simulink model "MIL4L3_SW6_V1_20220211"  (R2018b)
settings: Solver=FixedStepAuto  StartTime=0.0  StopTime=inf  FixedStep=0.001  RelTol=1e-3
PreLoadFcn:
  | A0_MILtest;
undefined symbols (not defined in the file or in its folder): Clb_ICADirect_LaneDisp_StateFive, Clb_ICADirect_LaneDisp_StateFour, Clb_ICADirect_LaneDisp_StateOne, Clb_ICADirect_LaneDisp_StateThree, Clb_ICADirect_LaneDisp_StateTwo, Clb_ICADirect_LaneDisp_StateZero, Clb_ICADirect_LaneDispSW, Clb_ICADirect_TrnLghtsCom_Switch, Clb_ICADirect_TrnLghtsCom_Value, Clb_ICADirect_TrnLghtsCrtl_Inhb, IMAP_Clb_ACU_Driver_Belt, IMAP_Clb_ACU_Driver_Belt_Over, IMAP_Clb_ACU_Passenger_Belt, IMAP_Clb_ACU_Passenger_Belt_Over, IMAP_Clb_ACU_RearLeft_Belt, IMAP_Clb_ACU_RearLeft_Belt_Over, IMAP_Clb_ACU_RearMiddle_Belt, IMAP_Clb_ACU_RearMiddle_Belt_Over, IMAP_Clb_ACU_RearRight_Belt, IMAP_Clb_ACU_RearRight_Belt_Over, IMAP_Clb_AEB_Switch, IMAP_Clb_AEB_Switch_Over, IMAP_Clb_ALC_TLC_Mode, IMAP_Clb_ALC_TLC_Mode_Over, IMAP_Clb_BCM_Battery_Voltage, IMAP_Clb_BCM_Battery_Voltage_Over, IMAP_Clb_BCM_BrakeLamp_State, IMAP_Clb_BCM_BrakeLamp_State_Over, IMAP_Clb_BCM_CHMSL_Status, IMAP_Clb_BCM_CHMSL_Status_Over, IMAP_Clb_BCM_Door_Lock_State, IMAP_Clb_BCM_Door_Lock_State_Over, IMAP_Clb_BCM_FrontWiper_State, IMAP_Clb_BCM_FrontWiper_State_Over, IMAP_Clb_BCM_FrontWiper_Switch, IMAP_Clb_BCM_FrontWiper_Switch_Over, IMAP_Clb_BCM_HazardLamp, IMAP_Clb_BCM_HazardLamp_Over, IMAP_Clb_BCM_HazardLamp_Switch, IMAP_Clb_BCM_HazardLamp_Switch_Over, IMAP_Clb_BCM_HighBeam_State, IMAP_Clb_BCM_HighBeam_State_Over, IMAP_Clb_BCM_Ignition_State, IMAP_Clb_BCM_Ignition_State_Over, IMAP_Clb_BCM_IHBC_Enabled, IMAP_Clb_BCM_IHBC_Enabled_Over, IMAP_Clb_BCM_Left_Light, IMAP_Clb_BCM_Left_Light_Over, IMAP_Clb_BCM_LeftTurn_Switch, IMAP_Clb_BCM_LeftTurn_Switch_Over, IMAP_Clb_BCM_LF_Door_State, IMAP_Clb_BCM_LF_Door_State_Over, IMAP_Clb_BCM_LowBeam_State, IMAP_Clb_BCM_LowBeam_State_Over, IMAP_Clb_BCM_LR_Door_State, IMAP_Clb_BCM_LR_Door_State_Over, IMAP_Clb_BCM_RF_Door_State, IMAP_Clb_BCM_RF_Door_State_Over, IMAP_Clb_BCM_Right_Light, IMAP_Clb_BCM_Right_Light_Over ... (+547)
libraries: CarMaker4SL x2153, simulink x292, dspstat3 x3, canmsglib x2, simulink_extras x1
(part 7 of 52)

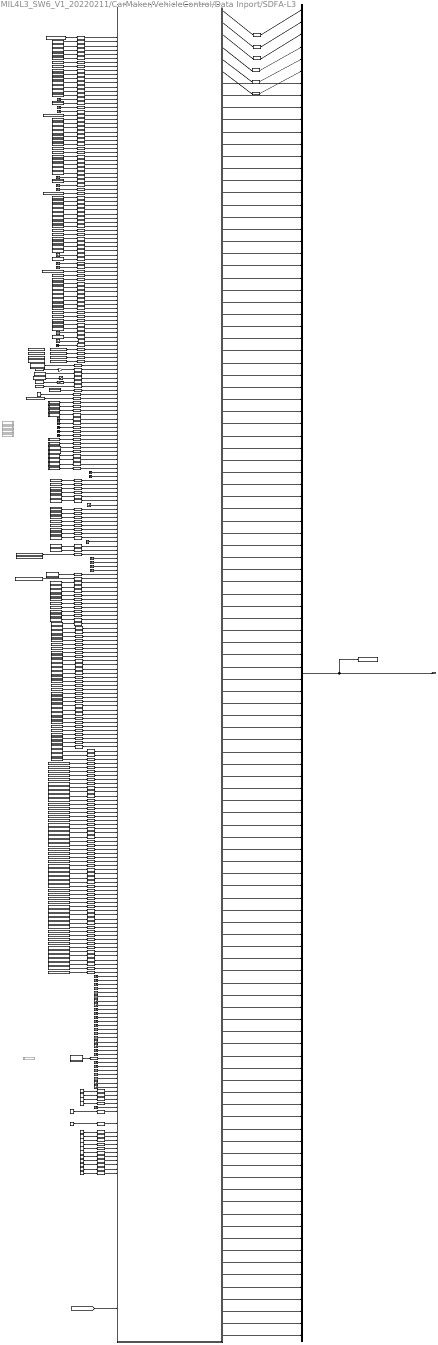
== system MIL4L3_SW6_V1_20220211/CarMaker/VehicleControl/Data Inport/SDFA-L3 ==
  note: SDFA-L3
  ACCEL_LONGI_CALIB2 : Saturate  UpperLimit=40.92  LowerLimit=-40.96
  BusCreator3 : BusCreator  Inputs=110
  CIPV_ID1 : Subsystem
  Constant{1..8,10..14,16..19} (17 alike) : Constant  Value=0
  Constant9 : Constant
  Data Type  Conversion{1..4,6,8..12,508} (11 alike) : DataTypeConversion
  Data Type Conversion{,1..94,98,118,128..129,131..251,253..265,267} (234 alike) : DataTypeConversion
  Define CM Dict : CarMaker4SL/Define CM Dict  xname=User.IO.Out.CRFLstatus  xmono=off  xtype=Double4  xdvaplace=None  xnstates=0  xfirststate=0  xinitial=0
  Define CM Dict1 : CarMaker4SL/Define CM Dict  xname=User.IO.Out.CRFRstatus  xmono=off  xtype=Double4  xdvaplace=None  xnstates=0  xfirststate=0  xinitial=0
  Define CM Dict3 : CarMaker4SL/Define CM Dict  xname=User.IO.Out.CRRLstatus  xmono=off  xtype=Double4  xdvaplace=None  xnstates=0  xfirststate=0  xinitial=0
  Define CM Dict4 : CarMaker4SL/Define CM Dict  xname=User.IO.Out.CRRRstatus  xmono=off  xtype=Double4  xdvaplace=None  xnstates=0  xfirststate=0  xinitial=0
  Define CM Dict7 : CarMaker4SL/Define CM Dict  xname=User.IO.Out.IFCState  xmono=off  xtype=Double4  xdvaplace=IO_Out  xnstates=0  xfirststate=0  xinitial=9
  Gain10 : Gain  Gain=3.6
  Ground{,1..41,43..46,52,56..61} (53 alike) : Ground
  Lateral_acceleration1 : CarMaker4SL/Read CM Dict  xname=Car.ay  xsync=off
  Lateral_acceleration2 : CarMaker4SL/Read CM Dict  xname=User.IO.Out.CRFLstatus  xsync=off
  Lateral_acceleration3 : CarMaker4SL/Read CM Dict  xname=User.IO.Out.CRFRstatus  xsync=off
  Lateral_acceleration4 : CarMaker4SL/Read CM Dict  xname=User.IO.Out.CRRLstatus  xsync=off
  Lateral_acceleration5 : CarMaker4SL/Read CM Dict  xname=User.IO.Out.CRRRstatus  xsync=off
  Read CM Dict : CarMaker4SL/Read CM Dict  xname=User.IO.Out.IFC_Line01_CurvChange  xsync=off
  Read CM Dict1 : CarMaker4SL/Read CM Dict  xname=User.IO.Out.NumberOfObjects_S3  xsync=off
  Read CM Dict10 : CarMaker4SL/Read CM Dict  xname=User.IO.Out.IFC_Line01_Dy  xsync=off
  Read CM Dict11 : CarMaker4SL/Read CM Dict  xname=User.IO.Out.IFC_Line01_ExistProb  xsync=off
  Read CM Dict12 : CarMaker4SL/Read CM Dict  xname=User.IO.Out.IFC_Line01_MeasureType  xsync=off
  Read CM Dict13 : CarMaker4SL/Read CM Dict  xname=User.IO.Out.IFC_Line01_Type  xsync=off
  Read CM Dict14 : CarMaker4SL/Read CM Dict  xname=User.IO.Out.IFC_Line01_LineID  xsync=off
  Read CM Dict15 : CarMaker4SL/Read CM Dict  xname=User.IO.Out.IFC_Line01_TypeConf  xsync=off
  Read CM Dict16 : CarMaker4SL/Read CM Dict  xname=User.IO.Out.IFC_Line01_ColorClass  xsync=off
  Read CM Dict17 : CarMaker4SL/Read CM Dict  xname=User.IO.Out.IFC_Line01_DxStart  xsync=off
  Read CM Dict18 : CarMaker4SL/Read CM Dict  xname=User.IO.Out.IFC_Line01_DxEnd  xsync=off
  Read CM Dict19 : CarMaker4SL/Read CM Dict  xname=User.IO.Out.IFC_Line01_LineWidth  xsync=off
  Read CM Dict2 : CarMaker4SL/Read CM Dict  xname=User.IO.Out.IFCState  xsync=off
  Read CM Dict20 : CarMaker4SL/Read CM Dict  xname=User.IO.Out.IFC_Line02_CurvChange  xsync=off
  Read CM Dict21 : CarMaker4SL/Read CM Dict  xname=User.IO.Out.IFC_Line02_Curv  xsync=off
  Read CM Dict22 : CarMaker4SL/Read CM Dict  xname=User.IO.Out.IFC_Line02_HeadingAngle  xsync=off
  Read CM Dict23 : CarMaker4SL/Read CM Dict  xname=User.IO.Out.IFC_Line02_Dy  xsync=off
  Read CM Dict24 : CarMaker4SL/Read CM Dict  xname=User.IO.Out.IFC_Line02_ExistProb  xsync=off
  Read CM Dict25 : CarMaker4SL/Read CM Dict  xname=Car.ax  xsync=off
  Read CM Dict26 : CarMaker4SL/Read CM Dict  xname=Car.v  xsync=off
  Read CM Dict27 : CarMaker4SL/Read CM Dict  xname=Steer.WhlAng  xsync=off
  Read CM Dict28 : CarMaker4SL/Read CM Dict  xname=User.IO.Out.IFC_Line02_MeasureType  xsync=off
  Read CM Dict29 : CarMaker4SL/Read CM Dict  xname=User.IO.Out.IFC_Line02_Type  xsync=off
  Read CM Dict3 : CarMaker4SL/Read CM Dict  xname=User.IO.Out.NumberOfObjects_S0  xsync=off
  Read CM Dict30 : CarMaker4SL/Read CM Dict  xname=User.IO.Out.IFC_Line02_LineID  xsync=off
  Read CM Dict31 : CarMaker4SL/Read CM Dict  xname=User.IO.Out.IFC_Line02_TypeConf  xsync=off
  Read CM Dict32 : CarMaker4SL/Read CM Dict  xname=User.IO.Out.IFC_Line02_ColorClass  xsync=off
  Read CM Dict33 : CarMaker4SL/Read CM Dict  xname=User.IO.Out.IFC_Line02_DxStart  xsync=off
  Read CM Dict34 : CarMaker4SL/Read CM Dict  xname=User.IO.Out.IFC_Line02_DxEnd  xsync=off
  Read CM Dict35 : CarMaker4SL/Read CM Dict  xname=User.IO.Out.IFC_Line02_LineWidth  xsync=off
  Read CM Dict36 : CarMaker4SL/Read CM Dict  xname=User.IO.Out.IFC_Line03_CurvChange  xsync=off
  Read CM Dict37 : CarMaker4SL/Read CM Dict  xname=User.IO.Out.IFC_Line03_Curv  xsync=off
  Read CM Dict38 : CarMaker4SL/Read CM Dict  xname=User.IO.Out.IFC_Line03_HeadingAngle  xsync=off
  Read CM Dict39 : CarMaker4SL/Read CM Dict  xname=User.IO.Out.IFC_Line03_Dy  xsync=off
  Read CM Dict4 : CarMaker4SL/Read CM Dict  xname=User.IO.Out.NumberOfObjects_S1  xsync=off
  Read CM Dict40 : CarMaker4SL/Read CM Dict  xname=User.IO.Out.IFC_Line03_ExistProb  xsync=off
  Read CM Dict41 : CarMaker4SL/Read CM Dict  xname=User.IO.Out.IFC_Line03_MeasureType  xsync=off
  Read CM Dict42 : CarMaker4SL/Read CM Dict  xname=User.IO.Out.IFC_Line03_Type  xsync=off
  Read CM Dict43 : CarMaker4SL/Read CM Dict  xname=User.IO.Out.IFC_Line03_LineID  xsync=off
  Read CM Dict44 : CarMaker4SL/Read CM Dict  xname=User.IO.Out.IFC_Line03_TypeConf  xsync=off
  Read CM Dict45 : CarMaker4SL/Read CM Dict  xname=User.IO.Out.IFC_Line03_ColorClass  xsync=off
  Read CM Dict46 : CarMaker4SL/Read CM Dict  xname=User.IO.Out.IFC_Line03_DxStart  xsync=off
  Read CM Dict47 : CarMaker4SL/Read CM Dict  xname=User.IO.Out.IFC_Line03_DxEnd  xsync=off
  Read CM Dict48 : CarMaker4SL/Read CM Dict  xname=User.IO.Out.IFC_Line03_LineWidth  xsync=off
  Read CM Dict49 : CarMaker4SL/Read CM Dict  xname=User.IO.Out.IFC_Line04_CurvChange  xsync=off
  Read CM Dict5 : CarMaker4SL/Read CM Dict  xname=User.IO.Out.NumberOfObjects_S2  xsync=off
  Read CM Dict50 : CarMaker4SL/Read CM Dict  xname=User.IO.Out.IFC_Line04_Curv  xsync=off
  Read CM Dict51 : CarMaker4SL/Read CM Dict  xname=User.IO.Out.IFC_Line04_HeadingAngle  xsync=off
  Read CM Dict52 : CarMaker4SL/Read CM Dict  xname=User.IO.Out.IFC_Line04_Dy  xsync=off
  Read CM Dict53 : CarMaker4SL/Read CM Dict  xname=User.IO.Out.IFC_Line04_ExistProb  xsync=off
  Read CM Dict54 : CarMaker4SL/Read CM Dict  xname=User.IO.Out.IFC_Line04_MeasureType  xsync=off
  Read CM Dict55 : CarMaker4SL/Read CM Dict  xname=User.IO.Out.IFC_Line04_Type  xsync=off
  Read CM Dict56 : CarMaker4SL/Read CM Dict  xname=User.IO.Out.IFC_Line04_LineID  xsync=off
  Read CM Dict57 : CarMaker4SL/Read CM Dict  xname=User.IO.Out.IFC_Line04_TypeConf  xsync=off
  Read CM Dict58 : CarMaker4SL/Read CM Dict  xname=User.IO.Out.IFC_Line04_ColorClass  xsync=off
  Read CM Dict59 : CarMaker4SL/Read CM Dict  xname=User.IO.Out.IFC_Line04_DxStart  xsync=off
  Read CM Dict6 : CarMaker4SL/Read CM Dict  xname=User.IO.Out.NumberOfObj  xsync=off
  Read CM Dict60 : CarMaker4SL/Read CM Dict  xname=User.IO.Out.IFC_Line04_DxEnd  xsync=off
  Read CM Dict61 : CarMaker4SL/Read CM Dict  xname=User.IO.Out.IFC_Line04_LineWidth  xsync=off
  Read CM Dict62 : CarMaker4SL/Read CM Dict  xname=User.IO.Out.ObjCount  xsync=off
  Read CM Dict8 : CarMaker4SL/Read CM Dict  xname=User.IO.Out.IFC_Line01_Curv  xsync=off
  Read CM Dict9 : CarMaker4SL/Read CM Dict  xname=User.IO.Out.IFC_Line01_HeadingAngle  xsync=off
  SDFA-L3 : ModelReference  ModelNameDialog=SDFA_SW6_1_MIL.slxp  ModelReferenceVersion=1.248  CopyOfModelProtected=on
  Saturation3 : Saturate  UpperLimit=780  LowerLimit=-780
  Subsystem : Subsystem
  Subsystem1 : Subsystem
  Subsystem10 : Subsystem
  Subsystem100 : Subsystem
  Subsystem103 : Subsystem
  Subsystem107 : Subsystem
  Subsystem108 : Subsystem
  Subsystem109 : Subsystem
  Subsystem11 : Subsystem
  Subsystem110 : Subsystem
  Subsystem111 : Subsystem
  Subsystem112 : Subsystem
  Subsystem113 : Subsystem
  Subsystem114 : Subsystem
  Subsystem115 : Subsystem
  Subsystem116 : Subsystem
  Subsystem117 : Subsystem
  Subsystem118 : Subsystem
  Subsystem119 : Subsystem
  Subsystem12 : Subsystem
  Subsystem120 : Subsystem
  Subsystem14 : Subsystem
  Subsystem149 : Subsystem
  Subsystem150 : Subsystem
  Subsystem160 : Subsystem
  Subsystem171 : Subsystem
  Subsystem174 : Subsystem
  Subsystem175 : Subsystem
  Subsystem176 : Subsystem
  Subsystem177 : Subsystem
  Subsystem178 : Subsystem
  Subsystem179 : Subsystem
  Subsystem180 : Subsystem
  Subsystem181 : Subsystem
  Subsystem182 : Subsystem
  Subsystem183 : Subsystem
  Subsystem184 : Subsystem
  Subsystem185 : Subsystem
  Subsystem186 : Subsystem
  Subsystem187 : Subsystem
  Subsystem188 : Subsystem
  Subsystem189 : Subsystem
  Subsystem190 : Subsystem
  Subsystem191 : Subsystem
  Subsystem192 : Subsystem
  Subsystem193 : Subsystem
  Subsystem194 : Subsystem
  Subsystem195 : Subsystem
  Subsystem196 : Subsystem
  Subsystem197 : Subsystem
  Subsystem198 : Subsystem
  Subsystem199 : Subsystem
  Subsystem2 : Subsystem
  Subsystem20 : Subsystem
  Subsystem200 : Subsystem
  Subsystem201 : Subsystem
  Subsystem202 : Subsystem
  Subsystem203 : Subsystem
  Subsystem204 : Subsystem
  Subsystem205 : Subsystem
  Subsystem206 : Subsystem
  Subsystem208 : Subsystem
  Subsystem209 : Subsystem
  Subsystem210 : Subsystem
  Subsystem211 : Subsystem
  Subsystem212 : Subsystem
  Subsystem214 : Subsystem
  Subsystem215 : Subsystem
  Subsystem216 : Subsystem
  Subsystem217 : Subsystem
  Subsystem218 : Subsystem
  Subsystem219 : Subsystem
  Subsystem220 : Subsystem
  Subsystem221 : Subsystem
  Subsystem222 : Subsystem
  Subsystem223 : Subsystem
  Subsystem224 : Subsystem
  Subsystem225 : Subsystem
  Subsystem226 : Subsystem
  Subsystem227 : Subsystem
  Subsystem228 : Subsystem
  Subsystem230 : Subsystem  Commented=on
  Subsystem232 : Subsystem
  Subsystem239 : Subsystem  Commented=on
  Subsystem255 : Subsystem
  Subsystem261 : Subsystem  Commented=on
  Subsystem272 : Subsystem  Commented=on
  Subsystem283 : Subsystem
  Subsystem3 : Subsystem
  Subsystem4 : Subsystem
  Subsystem40 : Subsystem
  Subsystem41 : Subsystem  Commented=on
  Subsystem46 : Subsystem
  Subsystem47 : Subsystem
  Subsystem48 : Subsystem
  Subsystem49 : Subsystem
  Subsystem5 : Subsystem
  Subsystem50 : Subsystem
  Subsystem51 : Subsystem
  Subsystem52 : Subsystem
  Subsystem53 : Subsystem
  Subsystem54 : Subsystem
  Subsystem55 : Subsystem
  Subsystem56 : Subsystem
  Subsystem57 : Subsystem
  Subsystem58 : Subsystem
  Subsystem59 : Subsystem
  Subsystem6 : Subsystem
  Subsystem61 : Subsystem
  Subsystem66 : Subsystem
  Subsystem67 : Subsystem
  Subsystem68 : Subsystem
  Subsystem69 : Subsystem
  Subsystem7 : Subsystem
  Subsystem70 : Subsystem
  Subsystem71 : Subsystem
  Subsystem72 : Subsystem
  Subsystem73 : Subsystem
  Subsystem74 : Subsystem
  Subsystem75 : Subsystem
  Subsystem76 : Subsystem
  Subsystem77 : Subsystem
  Subsystem78 : Subsystem
  Subsystem79 : Subsystem
  Subsystem8 : Subsystem
  Subsystem81 : Subsystem
  Subsystem85 : Subsystem
  Subsystem86 : Subsystem
  Subsystem87 : Subsystem
  Subsystem88 : Subsystem
  Subsystem89 : Subsystem
  Subsystem9 : Subsystem
  Subsystem90 : Subsystem
  Subsystem91 : Subsystem
  Subsystem92 : Subsystem
  Subsystem93 : Subsystem
  Subsystem94 : Subsystem
  Subsystem95 : Subsystem
  Subsystem96 : Subsystem
  Subsystem97 : Subsystem
  Subsystem98 : Subsystem
  To Workspace : ToWorkspace  VariableName=SDFAOUTPUT  SaveFormat=Timeseries  SampleTime=-1
  SDFAL3 : Outport
  wires:
  BusCreator3/1 -> To Workspace/1, SDFAL3/1
  SDFA-L3/1 -> Data Type  Conversion8/1
  SDFA-L3/6 -> Data Type  Conversion4/1
  Data Type  Conversion10/1 -> BusCreator3/3  "SDFAve_d_sen_sta_RF_radar"
  SDFA-L3/2 -> Data Type  Conversion9/1
  Data Type  Conversion9/1 -> BusCreator3/2  "SDFAve_d_sen_sta_LF_radar"
  Data Type  Conversion8/1 -> BusCreator3/1  "SDFAve_d_sensor_status"
  Data Type  Conversion11/1 -> BusCreator3/4  "SDFAve_d_sen_sta_LB_radar"
  Data Type  Conversion12/1 -> BusCreator3/5  "SDFAve_d_sen_sta_RB_radar"
  SDFA-L3/3 -> Data Type  Conversion10/1
  SDFA-L3/4 -> Data Type  Conversion11/1
  SDFA-L3/5 -> Data Type  Conversion12/1
  Lateral_acceleration2/1 -> Data Type Conversion131/1
  Lateral_acceleration3/1 -> Data Type Conversion132/1
  Lateral_acceleration4/1 -> Data Type Conversion133/1
  Lateral_acceleration5/1 -> Data Type Conversion134/1
  Data Type Conversion131/1 -> SDFA-L3/77
  Data Type Conversion132/1 -> SDFA-L3/78
  Data Type Conversion133/1 -> SDFA-L3/79
  Data Type Conversion134/1 -> SDFA-L3/80
  Data Type  Conversion4/1 -> BusCreator3/6  "SDFAve_d_fusion_status"
  Data Type Conversion149/1 -> SDFA-L3/12  "LFtar_ExistenceProbability"
  Data Type Conversion145/1 -> SDFA-L3/8  "LFtar_Yacceleration"
  Data Type Conversion148/1 -> SDFA-L3/11  "LFtar_Orientation"
  Data Type Conversion186/1 -> SDFA-L3/51  "LBtar_Class"
  Data Type Conversion139/1 -> SDFA-L3/2  "LFtar_id"
  Data Type Conversion206/1 -> SDFA-L3/73  "RBtar_ObjectInfo"
  Data Type Conversion150/1 -> SDFA-L3/13  "LFtar_Class"
  Data Type Conversion178/1 -> SDFA-L3/44  "LBtar_Yvelocity"
  Data Type Conversion179/1 -> SDFA-L3/45  "LBtar_Xacceleration"
  Data Type Conversion177/1 -> SDFA-L3/43  "LBtar_Xvelocity"
  Data Type Conversion167/1 -> SDFA-L3/32  "RFtar_Class"
  Data Type Conversion187/1 -> SDFA-L3/52  "LBtar_ReferencePoint"
  Data Type Conversion151/1 -> SDFA-L3/14  "LFtar_ReferencePoint"
  Data Type Conversion165/1 -> SDFA-L3/30  "RFtar_Orientation"
  Data Type Conversion147/1 -> SDFA-L3/10  "LFtar_Length"
  Data Type Conversion164/1 -> SDFA-L3/29  "RFtar_Length"
  Data Type Conversion163/1 -> SDFA-L3/28  "RFtar_Width"
  Data Type Conversion162/1 -> SDFA-L3/27  "RFtar_Yacceleration"
  Data Type Conversion161/1 -> SDFA-L3/26  "RFtar_Xacceleration"
  Data Type Conversion170/1 -> SDFA-L3/36  "RFtar_ClassHighestProb"
  Data Type Conversion169/1 -> SDFA-L3/35  "RFtar_ObjectInfo"
  Data Type Conversion188/1 -> SDFA-L3/54  "LBtar_ObjectInfo"
  Data Type Conversion193/1 -> SDFA-L3/61  "RBtar_Ypos"
  Data Type Conversion191/1 -> SDFA-L3/58  "RBtar_number"
  Data Type Conversion194/1 -> SDFA-L3/60  "RBtar_Xpos"
  Data Type Conversion143/1 -> SDFA-L3/6  "LFtar_Yvelocity"
  Subsystem47/1(LFtar_Xpos) -> Data Type Conversion140/1  "LFtar_Xpos"
  Data Type Conversion158/1 -> SDFA-L3/16  "LFtar_ObjectInfo"
  Subsystem46/1(LFtar_id) -> Data Type Conversion139/1  "LFtar_id"
  Data Type Conversion138/1 -> SDFA-L3/1  "LFtar_number"
  Data Type Conversion181/1 -> SDFA-L3/47  "LBtar_Width"
  Data Type Conversion184/1 -> SDFA-L3/50  "LBtar_ExistenceProbability"
  Data Type Conversion160/1 -> SDFA-L3/25  "RFtar_Yvelocity"
  Data Type Conversion197/1 -> SDFA-L3/63  "RBtar_Yvelocity"
  Data Type Conversion200/1 -> SDFA-L3/65  "RBtar_Yacceleration"
  Data Type Conversion182/1 -> SDFA-L3/48  "LBtar_Length"
  Data Type Conversion199/1 -> SDFA-L3/66  "RBtar_Width"
  Data Type Conversion203/1 -> SDFA-L3/69  "RBtar_ExistenceProbability"
  Data Type Conversion202/1 -> SDFA-L3/68  "RBtar_Orientation"
  Data Type Conversion189/1 -> SDFA-L3/55  "LBtar_ClassHighestProb"
  Data Type Conversion144/1 -> SDFA-L3/7  "LFtar_Xacceleration"
  Data Type Conversion140/1 -> SDFA-L3/3  "LFtar_Xpos"
  Data Type Conversion168/1 -> SDFA-L3/33  "RFtar_ReferencePoint"
  Data Type Conversion192/1 -> SDFA-L3/59  "RBtar_id"
  Data Type Conversion171/1 -> SDFA-L3/38  "RFtar_timestamp"
  Data Type Conversion208/1 -> SDFA-L3/74  "RBtar_ClassHighestProb"
  Data Type Conversion176/1 -> SDFA-L3/42  "LBtar_Ypos"
  Data Type Conversion172/1 -> SDFA-L3/39  "LBtar_number"
  Data Type Conversion142/1 -> SDFA-L3/5  "LFtar_Xvelocity"
  Data Type Conversion141/1 -> SDFA-L3/4  "LFtar_Ypos"
  Data Type Conversion166/1 -> SDFA-L3/31  "RFtar_ExistenceProbability"
  Data Type Conversion173/1 -> SDFA-L3/40  "LBtar_id"
  Data Type Conversion175/1 -> SDFA-L3/41  "LBtar_Xpos"
  Data Type Conversion201/1 -> SDFA-L3/67  "RBtar_Length"
  Data Type Conversion205/1 -> SDFA-L3/70  "RBtar_Class"
  Data Type Conversion204/1 -> SDFA-L3/71  "RBtar_ReferencePoint"
  Data Type Conversion152/1 -> SDFA-L3/19  "LFtar_timestamp"
  Data Type Conversion198/1 -> SDFA-L3/64  "RBtar_Xacceleration"
  Data Type Conversion154/1 -> SDFA-L3/21  "RFtar_id"
  Data Type Conversion156/1 -> SDFA-L3/23  "RFtar_Ypos"
  Data Type Conversion185/1 -> SDFA-L3/15  "LFtar_MovingState"
  Subsystem70/1(RFtar_Yvelocity) -> Data Type Conversion160/1  "RFtar_Yvelocity"
  Data Type Conversion155/1 -> SDFA-L3/22  "RFtar_Xpos"
  Data Type Conversion137/1 -> SDFA-L3/75  "RBtar_MessageCounter"
  Ground40/1 -> Data Type Conversion171/1  "RFtar_timestamp"
  Data Type Conversion159/1 -> SDFA-L3/17  "LFtar_ClassHighestProb"
  Data Type Conversion210/1 -> SDFA-L3/53  "LBtar_MovingState"
  Data Type Conversion136/1 -> SDFA-L3/72  "RBtar_MovingState"
  Data Type Conversion135/1 -> SDFA-L3/56  "LBtar_MessageCounter"
  Data Type Conversion207/1 -> SDFA-L3/37  "RFtar_MessageCounter"
  Data Type Conversion196/1 -> SDFA-L3/34  "RFtar_MovingState"
  Subsystem85/1(LBtar_id) -> Data Type Conversion173/1  "LBtar_id"
  Ground18/1 -> Data Type Conversion206/1  "RBtar_ObjectInfo"
  Data Type Conversion183/1 -> SDFA-L3/49  "LBtar_Orientation"
  Subsystem78/1(RFtar_ReferencePoint) -> Data Type Conversion168/1  "RFtar_ReferencePoint"
  Subsystem61/1(LFtar_ClassHighestProb) -> Data Type Conversion159/1  "LFtar_ClassHighestProb"
  Subsystem59/1(LFtar_MovingState) -> Data Type Conversion185/1
  Subsystem48/1(LFtar_Ypos) -> Data Type Conversion141/1  "LFtar_Ypos"
  Subsystem53/1(LFtar_Width) -> Data Type Conversion146/1  "LFtar_Width"
  Read CM Dict5/1 -> Data Type Conversion138/1
  Subsystem67/1(RFtar_Xpos) -> Data Type Conversion155/1  "RFtar_Xpos"
  Subsystem50/1(LFtar_Yvelocity) -> Data Type Conversion143/1  "LFtar_Yvelocity"
  Subsystem94/1(LBtar_Orientation) -> Data Type Conversion183/1  "LBtar_Orientation"
  Subsystem117/1(RBtar_ExistenceProbability) -> Data Type Conversion203/1  "RBtar_ExistenceProbability"
  Subsystem68/1(RFtar_Ypos) -> Data Type Conversion156/1  "RFtar_Ypos"
  Subsystem88/1(LBtar_Xvelocity) -> Data Type Conversion177/1  "LBtar_Xvelocity"
  Subsystem114/1(RBtar_Width) -> Data Type Conversion199/1  "RBtar_Width"
  Subsystem76/1(RFtar_ExistenceProbability) -> Data Type Conversion166/1  "RFtar_ExistenceProbability"
  Subsystem110/1(RBtar_Xvelocity) -> Data Type Conversion195/1  "RBtar_Xvelocity"
  Ground41/1 -> Data Type Conversion207/1
  Subsystem51/1(LFtar_Xacceleration) -> Data Type Conversion144/1  "LFtar_Xacceleration"
  Subsystem58/1(LFtar_ReferencePoint) -> Data Type Conversion151/1  "LFtar_ReferencePoint"
  Subsystem90/1(LBtar_Xacceleration) -> Data Type Conversion179/1  "LBtar_Xacceleration"
  Data Type Conversion146/1 -> SDFA-L3/9  "LFtar_Width"
  Subsystem87/1(LBtar_Ypos) -> Data Type Conversion176/1  "LBtar_Ypos"
  Ground45/1 -> Data Type Conversion135/1
  Data Type Conversion153/1 -> SDFA-L3/20  "RFtar_number"
  Ground17/1 -> Data Type Conversion152/1  "LFtar_timestamp"
  Ground29/1 -> Data Type Conversion190/1  "LBtar_timestamp"
  Subsystem77/1(RFtar_Class) -> Data Type Conversion167/1  "RFtar_Class"
  Read CM Dict4/1 -> Data Type Conversion191/1  "RBtar_number"
  Subsystem74/1(RFtar_Length) -> Data Type Conversion164/1  "RFtar_Length"
  Subsystem52/1(LFtar_Yacceleration) -> Data Type Conversion145/1  "LFtar_Yacceleration"
  Ground20/1 -> Data Type Conversion209/1  "RBtar_timestamp"
  Subsystem69/1(RFtar_Xvelocity) -> Data Type Conversion157/1  "RFtar_Xvelocity"
  Data Type Conversion190/1 -> SDFA-L3/57  "LBtar_timestamp"
  Subsystem55/1(LFtar_Orientation) -> Data Type Conversion148/1  "LFtar_Orientation"
  Subsystem100/1(LBtar_ClassHighestProb) -> Data Type Conversion189/1  "LBtar_ClassHighestProb"
  Subsystem89/1(LBtar_Yvelocity) -> Data Type Conversion178/1  "LBtar_Yvelocity"
  Subsystem109/1(RBtar_Ypos) -> Data Type Conversion193/1  "RBtar_Ypos"
  Ground46/1 -> Data Type Conversion137/1
  Subsystem119/1(RBtar_ReferencePoint) -> Data Type Conversion204/1  "RBtar_ReferencePoint"
  Subsystem49/1(LFtar_Xvelocity) -> Data Type Conversion142/1  "LFtar_Xvelocity"
  Subsystem92/1(LBtar_Width) -> Data Type Conversion181/1  "LBtar_Width"
  Read CM Dict3/1 -> Data Type Conversion172/1  "LBtar_number"
  Subsystem96/1(LBtar_Class) -> Data Type Conversion186/1  "LBtar_Class"
  Subsystem66/1(RFtar_id) -> Data Type Conversion154/1  "RFtar_id"
  Subsystem72/1(RFtar_Yacceleration) -> Data Type Conversion162/1  "RFtar_Yacceleration"
  Subsystem120/1(RBtar_MovingState) -> Data Type Conversion136/1
  Subsystem118/1(RBtar_Class) -> Data Type Conversion205/1  "RBtar_Class"
  Subsystem79/1(RFtar_MovingState) -> Data Type Conversion196/1
  Data Type Conversion174/1 -> SDFA-L3/18  "LFtar_MessageCounter"
  Subsystem107/1(RBtar_id) -> Data Type Conversion192/1  "RBtar_id"
  Subsystem95/1(LBtar_ExistenceProbability) -> Data Type Conversion184/1  "LBtar_ExistenceProbability"
  Subsystem81/1(RFtar_ClassHighestProb) -> Data Type Conversion170/1  "RFtar_ClassHighestProb"
  Subsystem116/1(RBtar_Orientation) -> Data Type Conversion202/1  "RBtar_Orientation"
  Subsystem111/1(RBtar_Yvelocity) -> Data Type Conversion197/1  "RBtar_Yvelocity"
  Ground15/1 -> Data Type Conversion174/1
  Subsystem54/1(LFtar_Length) -> Data Type Conversion147/1  "LFtar_Length"
  Subsystem56/1(LFtar_ExistenceProbability) -> Data Type Conversion149/1  "LFtar_ExistenceProbability"
  Subsystem86/1(LBtar_Xpos) -> Data Type Conversion175/1  "LBtar_Xpos"
  Subsystem75/1(RFtar_Orientation) -> Data Type Conversion165/1  "RFtar_Orientation"
  Subsystem57/1(LFtar_Class) -> Data Type Conversion150/1  "LFtar_Class"
  Data Type Conversion195/1 -> SDFA-L3/62  "RBtar_Xvelocity"
  Ground22/1 -> Data Type Conversion188/1  "LBtar_ObjectInfo"
  Subsystem115/1(RBtar_Length) -> Data Type Conversion201/1  "RBtar_Length"
  Subsystem108/1(RBtar_Xpos) -> Data Type Conversion194/1  "RBtar_Xpos"
  Ground14/1 -> Data Type Conversion158/1  "LFtar_ObjectInfo"
  Subsystem98/1(LBtar_MovingState) -> Data Type Conversion210/1
  Read CM Dict1/1 -> Data Type Conversion153/1  "RFtar_number"
  Subsystem112/1(RBtar_Xacceleration) -> Data Type Conversion198/1  "RBtar_Xacceleration"
  Data Type Conversion157/1 -> SDFA-L3/24  "RFtar_Xvelocity"
  Ground38/1 -> Data Type Conversion169/1  "RFtar_ObjectInfo"
  Subsystem97/1(LBtar_ReferencePoint) -> Data Type Conversion187/1  "LBtar_ReferencePoint"
  Subsystem73/1(RFtar_Width) -> Data Type Conversion163/1  "RFtar_Width"
  Subsystem113/1(RBtar_Yacceleration) -> Data Type Conversion200/1  "RBtar_Yacceleration"
  Subsystem71/1(RFtar_Xacceleration) -> Data Type Conversion161/1  "RFtar_Xacceleration"
  Data Type Conversion180/1 -> SDFA-L3/46  "LBtar_Yacceleration"
  Subsystem91/1(LBtar_Yacceleration) -> Data Type Conversion180/1  "LBtar_Yacceleration"
  Subsystem103/1(RBtar_ClassHighestProb) -> Data Type Conversion208/1  "RBtar_ClassHighestProb"
  Subsystem93/1(LBtar_Length) -> Data Type Conversion182/1  "LBtar_Length"
  Data Type Conversion209/1 -> SDFA-L3/76  "RBtar_timestamp"
  Ground28/1 -> SDFA-L3/241  "IFC_Roaddge02_MessureType"
  Subsystem194/1(obj_DySTD) -> Data Type Conversion25/1
  Data Type Conversion16/1 -> SDFA-L3/164  "IFC_obj_WidthStdDev"
  Data Type Conversion7/1 -> SDFA-L3/102  "AbsoluteLongAccSTD"
  Ground61/1 -> SDFA-L3/108  "AbsAccCov"
  Subsystem283/1(AbsoluteLongVelo) -> Data Type Conversion262/1
  Read CM Dict14/1 -> Data Type Conversion56/1
  Read CM Dict40/1 -> Data Type Conversion228/1
  Ground26/1 -> SDFA-L3/239  "IFC_Roaddge01_LineID"
  Ground12/1 -> SDFA-L3/236  "IFC_Roaddge01_DxEnd"
  Data Type Conversion61/1 -> SDFA-L3/184  "IFC_Line01_Type"
  Ground33/1 -> SDFA-L3/252  "FS_Splashes_0"
  Read CM Dict21/1 -> Data Type Conversion68/1
  Data Type Conversion260/1 -> SDFA-L3/96  "RelativeLatVelo"
  Subsystem184/1(obj_PhiRightSTD) -> Data Type Conversion15/1
  Data Type Conversion223/1 -> SDFA-L3/204  "IFC_Line03_CurvChange"
  Data Type Conversion219/1 -> SDFA-L3/200  "IFC_Line02_ColorClass"
  Subsystem255/1(AbsoluteLongVeloSTD) -> Data Type Conversion6/1
  Read CM Dict11/1 -> Data Type Conversion58/1
  Data Type Conversion68/1 -> SDFA-L3/192  "IFC_Line02_Curv"
  Subsystem198/1(obj_Rel_VxSTD) -> Data Type Conversion29/1
  Ground2/1 -> SDFA-L3/248  "IFC_Roaddge02_ExistProb"
  Data Type Conversion230/1 -> SDFA-L3/210  "IFC_Line03_Type"
  Ground21/1 -> SDFA-L3/245  "IFC_Roaddge02_Dy"
  Read CM Dict61/1 -> Data Type Conversion251/1
  Ground16/1 -> SDFA-L3/238  "IFC_Roaddge01_ExistProb"
  Data Type Conversion25/1 -> SDFA-L3/152  "IFC_obj_DyStdDev"
  Ground30/1 -> SDFA-L3/242  "IFC_Roaddge02_CurvChange"
  Ground23/1 -> SDFA-L3/246  "IFC_Roaddge02_DxEnd"
  Data Type Conversion73/1 -> SDFA-L3/174  "IFC_obj_BrakeLight"
  Ground24/1 -> SDFA-L3/247  "IFC_Roaddge02_DxStart"
  Ground13/1 -> SDFA-L3/237  "IFC_Roaddge01_DxStart"
  Subsystem224/1(obj_Heading) -> Data Type Conversion49/1
  Ground11/1 -> SDFA-L3/235  "IFC_Roaddge01_Dy"
  Data Type Conversion259/1 -> SDFA-L3/97  "RelativeLatAcc"
  Data Type Conversion11/1 -> SDFA-L3/114  "WidhSTD"
  Ground1/1 -> SDFA-L3/230  "IFC_Roaddge01_Type"
  Subsystem160/1(obj_Rel_Vx) -> Data Type Conversion224/1
  Data Type Conversion38/1 -> SDFA-L3/153  "IFC_obj_PhiLeft"
  Subsystem227/1(obj_Measured) -> Data Type Conversion52/1
  Data Type Conversion261/1 -> SDFA-L3/95  "RelativeLongVelo"
  Subsystem181/1(HeightSTD) -> Data Type Conversion12/1
  Read CM Dict30/1 -> Data Type Conversion217/1
  Data Type Conversion40/1 -> SDFA-L3/117  "ObjectID"
  Gain10/1 -> Data Type  Conversion508/1  "Vehicle_speed_of_wheelsensor"
  Data Type Conversion265/1 -> SDFA-L3/88  "ObjectListQuali"
  Subsystem217/1(obj_TypeProb) -> Data Type Conversion1/1
  Data Type Conversion22/1 -> SDFA-L3/158  "IFC_obj_PhiBottomStdDev"
  CIPV_ID1/1(Out1) -> Data Type Conversion39/1  "CIVP_ID"
  Data Type Conversion56/1 -> SDFA-L3/185  "IFC_Line01_LineID"
  Data Type Conversion39/1 -> SDFA-L3/132  "IFC_VD_CIPV_ID"
  Data Type Conversion29/1 -> SDFA-L3/141  "IFC_obj_Rel_VxStdDev"
  Subsystem188/1(obj_LengthSTD) -> Data Type Conversion19/1
  Constant2/1 -> Data Type Conversion128/1
  Subsystem186/1(obj_abgle_rate_STD) -> Data Type Conversion17/1
  Data Type Conversion34/1 -> SDFA-L3/122  "MovementStatus"
  Data Type Conversion47/1 -> SDFA-L3/167  "IFC_obj_Length"
  Data Type Conversion78/1 -> SDFA-L3/157  "IFC_obj_PhiBottom"
  Data Type Conversion15/1 -> SDFA-L3/156  "IFC_obj_PhiRightStdDev"
  Ground56/1 -> SDFA-L3/128  "FS_Low_Sun_0"
  Subsystem209/1(Length) -> Data Type Conversion46/1
  Data Type Conversion31/1 -> SDFA-L3/160  "IFC_obj_angle_3DStdDev"
  Ground6/1 -> SDFA-L3/232  "IFC_Roaddge01_CurvChange"
  Read CM Dict15/1 -> Data Type Conversion62/1
  Data Type Conversion229/1 -> SDFA-L3/209  "IFC_Line03_MeasureType"
  Read CM Dict38/1 -> Data Type Conversion226/1
  Data Type Conversion14/1 -> SDFA-L3/121  "YawSTD"
  Subsystem182/1(AbsoluteLatVelo) -> Data Type Conversion256/1
  Read CM Dict33/1 -> Data Type Conversion220/1
  Data Type Conversion48/1 -> SDFA-L3/169  "IFC_obj_ID"
  Subsystem187/1(obj_HeightSTD) -> Data Type Conversion18/1
  Data Type Conversion1/1 -> SDFA-L3/135  "IFC_obj_TypePron"
  Data Type Conversion77/1 -> SDFA-L3/159  "IFC_obj_angle_3D"
  Data Type Conversion248/1 -> SDFA-L3/226  "IFC_Line04_ColorClass"
  Data Type Conversion10/1 -> SDFA-L3/112  "LengthSTD"
  Data Type Conversion244/1 -> SDFA-L3/223  "IFC_Line04_Type"
  Data Type Conversion238/1 -> SDFA-L3/217  "IFC_Line04_CurvChange"
  Data Type Conversion79/1 -> SDFA-L3/144  "IFC_obj_Rel_VyStdDevValid"
  Ground19/1 -> SDFA-L3/244  "IFC_Roaddge02_HeadingAngle"
  Read CM Dict8/1 -> Data Type Conversion54/1
  Data Type  Conversion508/1 -> SDFA-L3/82  "SWINve_g_ESC_VeSpd"
  Data Type Conversion262/1 -> SDFA-L3/99  "AbsoluteLongVelo"
  Data Type Conversion37/1 -> SDFA-L3/151  "IFC_obj_Dy"
  Data Type Conversion33/1 -> SDFA-L3/147  "IFC_obj_abs_Ay"
  Subsystem205/1(ClassType) -> Data Type Conversion254/1
  Data Type Conversion59/1 -> SDFA-L3/183  "IFC_Line01_MeasureType"
  Data Type Conversion12/1 -> SDFA-L3/116  "HeightSTD"
  Data Type Conversion236/1 -> SDFA-L3/215  "IFC_Line03_DxEnd"
  Subsystem193/1(obj_DxSTD) -> Data Type Conversion24/1
  Ground60/1 -> SDFA-L3/107  "AbsVeloCov"
  Data Type Conversion257/1 -> SDFA-L3/126  "ExistenceProb"
  Ground10/1 -> SDFA-L3/234  "IFC_Roaddge01_HeadingAngle"
  Ground27/1 -> SDFA-L3/240  "IFC_Roaddge02_Type"
  Read CM Dict39/1 -> Data Type Conversion227/1
  Data Type Conversion55/1 -> SDFA-L3/180  "IFC_Line01_HeadingAngle"
  Read CM Dict6/1 -> Data Type Conversion264/1
  Subsystem177/1(AbsoluteLatVeloSTD) -> Data Type Conversion8/1
  Data Type Conversion222/1 -> SDFA-L3/203  "IFC_Line02_LineWidth"
  Data Type Conversion263/1 -> SDFA-L3/98  "RelativeLongAcc"
  Data Type Conversion36/1 -> SDFA-L3/120  "YawAngle"
  Subsystem200/1(obj_abgle_3DSTD) -> Data Type Conversion31/1
  Data Type Conversion76/1 -> SDFA-L3/161  "IFC_obj_angle_rate"
  Data Type Conversion215/1 -> SDFA-L3/196  "IFC_Line02_MeasureType"
  Data Type Conversion20/1 -> SDFA-L3/172  "IFC_obj_HeadingStdDev"
  Data Type Conversion2/1 -> SDFA-L3/140  "IFC_obj_Rel_VyValid"
  Data Type Conversion49/1 -> SDFA-L3/171  "IFC_obj_Heading"
  Data Type Conversion243/1 -> SDFA-L3/222  "IFC_Line04_MeasureType"
  Data Type Conversion58/1 -> SDFA-L3/182  "IFC_Line01_ExistProb"
  Data Type Conversion63/1 -> SDFA-L3/187  "IFC_Line01_ColorClass"
  Data Type Conversion225/1 -> SDFA-L3/205  "IFC_Line03_Curv"
  Data Type Conversion46/1 -> SDFA-L3/111  "Length"
  Read CM Dict25/1 -> ACCEL_LONGI_CALIB2/1
  Data Type Conversion233/1 -> SDFA-L3/213  "IFC_Line03_ColorClass"
  Subsystem222/1(MeasurementStatus) -> Data Type Conversion32/1
  Read CM Dict31/1 -> Data Type Conversion218/1
  Data Type Conversion232/1 -> SDFA-L3/212  "LH_Lanemark_Type_Conf_03"
  Read CM Dict24/1 -> Data Type Conversion214/1
  Subsystem180/1(WidhSTD) -> Data Type Conversion11/1
  Read CM Dict10/1 -> Data Type Conversion57/1
  Ground58/1 -> SDFA-L3/130  "FS_Fog"
  Data Type Conversion28/1 -> SDFA-L3/148  "IFC_obj_abs_AyStdDev"
  Data Type Conversion35/1 -> SDFA-L3/149  "IFC_obj_Dx"
  Ground7/1 -> SDFA-L3/233  "IFC_Roaddge01_Curv"
  Data Type Conversion41/1 -> SDFA-L3/155  "IFC_obj_PhiRight"
  Subsystem226/1(obj_TTIPC) -> Data Type Conversion51/1
  Read CM Dict51/1 -> Data Type Conversion240/1
  Ground43/1 -> SDFA-L3/115  "Height"
  Subsystem214/1(obj_PhiRight) -> Data Type Conversion41/1
  Data Type Conversion66/1 -> SDFA-L3/190  "IFC_Line01_LineWidth"
  Data Type Conversion62/1 -> SDFA-L3/186  "LH_Lanemark_Type_Conf_01"
  Subsystem195/1(obj_PhiLeftSTD) -> Data Type Conversion26/1
  Read CM Dict19/1 -> Data Type Conversion66/1
  Subsystem203/1(obj_abs_Ax) -> Data Type Conversion23/1
  Data Type Conversion9/1 -> SDFA-L3/106  "AbsLatAccSTD"
  Ground/1 -> SDFA-L3/262  "IsNew"
  Data Type Conversion264/1 -> SDFA-L3/89  "NumberOfObj"
  Subsystem202/1(obj_Rel_VyValid) -> Data Type Conversion2/1
  Data Type  Conversion3/1 -> SDFA-L3/86  "SWINve_g_ESC_LateralAccelaration"
  Subsystem192/1(obj_Rel_Vy) -> Data Type Conversion246/1
  Data Type Conversion267/1 -> SDFA-L3/90  "LongDistance"
  Data Type Conversion227/1 -> SDFA-L3/207  "IFC_Line03_Dy"
  ACCEL_LONGI_CALIB2/1 -> Data Type  Conversion6/1  "ACCEL_LONGI_CALIB"
  Data Type Conversion24/1 -> SDFA-L3/150  "IFC_obj_DxStdDev"
  Ground31/1 -> SDFA-L3/243  "IFC_Roaddge02_Curv"
  Read CM Dict57/1 -> Data Type Conversion247/1
  Read CM Dict17/1 -> Data Type Conversion64/1
  Data Type Conversion27/1 -> SDFA-L3/146  "IFC_obj_abs_AxStdDev"
  Read CM Dict60/1 -> Data Type Conversion250/1
  Data Type Conversion246/1 -> SDFA-L3/139  "IFC_obj_Rel_Vy"
  Data Type Conversion234/1 -> SDFA-L3/214  "IFC_Line03_DxStart"
  Data Type Conversion253/1 -> SDFA-L3/110  "ClassProbValue"
  Read CM Dict13/1 -> Data Type Conversion61/1
  Data Type Conversion8/1 -> SDFA-L3/104  "AbsLatVeloSTD"
  Data Type Conversion81/1 -> SDFA-L3/125  "RadarCrossSection"
  Data Type Conversion3/1 -> SDFA-L3/92  "LatDistance"
  Read CM Dict58/1 -> Data Type Conversion248/1
  Subsystem183/1(YawSTD) -> Data Type Conversion14/1
  Data Type Conversion75/1 -> SDFA-L3/170  "IFC_obj_DirIndicator"
  Read CM Dict16/1 -> Data Type Conversion63/1
  Data Type Conversion216/1 -> SDFA-L3/197  "IFC_Line02_Type"
  Data Type Conversion247/1 -> SDFA-L3/225  "LH_Lanemark_Type_Conf_04"
  Read CM Dict45/1 -> Data Type Conversion233/1
  Data Type Conversion21/1 -> SDFA-L3/176  "IFC_obj_TTIPC_StdDev"
  Data Type Conversion217/1 -> SDFA-L3/198  "IFC_Line02_LineID"
  Data Type Conversion52/1 -> SDFA-L3/177  "IFC_obj_Measured"
  Read CM Dict47/1 -> Data Type Conversion236/1
  Read CM Dict46/1 -> Data Type Conversion234/1
  Subsystem150/1(AbsoluteLongAcc) -> Data Type Conversion258/1
  Data Type Conversion241/1 -> SDFA-L3/220  "IFC_Line04_Dy"
  Ground8/1 -> Data Type Conversion259/1
  Ground35/1 -> SDFA-L3/254  "FS_Partical_Blockage_0"
  Read CM Dict56/1 -> Data Type Conversion245/1
  Subsystem1/1(LongDistance) -> Data Type Conversion267/1
  Data Type Conversion220/1 -> SDFA-L3/201  "IFC_Line02_DxStart"
  Read CM Dict/1 -> Data Type Conversion53/1
  Read CM Dict9/1 -> Data Type Conversion55/1
  Subsystem176/1(AbsoluteLongAccSTD) -> Data Type Conversion7/1
  Read CM Dict23/1 -> Data Type Conversion212/1
  Data Type Conversion226/1 -> SDFA-L3/206  "IFC_Line03_HeadingAngle"
  Read CM Dict32/1 -> Data Type Conversion219/1
  Data Type Conversion240/1 -> SDFA-L3/219  "IFC_Line04_HeadingAngle"
  Ground44/1 -> SDFA-L3/124  "BrakingAllowed"
  Data Type Conversion26/1 -> SDFA-L3/154  "IFC_obj_PhiLeftStdDev"
  Subsystem215/1(ObjectID) -> Data Type Conversion40/1
  Read CM Dict59/1 -> Data Type Conversion249/1
  Ground5/1 -> Data Type Conversion260/1
  Read CM Dict54/1 -> Data Type Conversion243/1
  Subsystem219/1(YawAngle) -> Data Type Conversion36/1
  Data Type Conversion221/1 -> SDFA-L3/202  "IFC_Line02_DxEnd"
  Subsystem223/1(obj_ID) -> Data Type Conversion48/1
  Data Type Conversion70/1 -> SDFA-L3/118  "ObjectAge"
  Data Type Conversion5/1 -> SDFA-L3/93  "LateralDistanceSTD"
  Data Type Conversion258/1 -> SDFA-L3/101  "AbsoluteLongAcc"
  Data Type Conversion18/1 -> SDFA-L3/166  "IFC_obj_HeightStdDev"
  Ground9/1 -> Data Type Conversion263/1
  Subsystem196/1(obj_abs_AxSTD) -> Data Type Conversion27/1
  Read CM Dict28/1 -> Data Type Conversion215/1
  Read CM Dict29/1 -> Data Type Conversion216/1
  Read CM Dict42/1 -> Data Type Conversion230/1
  Read CM Dict52/1 -> Data Type Conversion241/1
  Saturation3/1 -> Data Type  Conversion2/1
  Subsystem189/1(obj_HeadingSTD) -> Data Type Conversion20/1
  Read CM Dict35/1 -> Data Type Conversion222/1
  Subsystem232/1(ClassProbValue) -> Data Type Conversion253/1
  Subsystem174/1(LateralDistanceSTD) -> Data Type Conversion5/1
  Read CM Dict43/1 -> Data Type Conversion231/1
  Data Type Conversion224/1 -> SDFA-L3/137  "IFC_obj_Rel_Vx"
  Read CM Dict18/1 -> Data Type Conversion65/1
  Subsystem175/1(LongDistanceSTD) -> Data Type Conversion4/1
  Data Type Conversion212/1 -> SDFA-L3/194  "IFC_Line02_Dy"
  Read CM Dict50/1 -> Data Type Conversion239/1
  Data Type Conversion218/1 -> SDFA-L3/199  "LH_Lanemark_Type_Conf_02"
  Data Type Conversion54/1 -> SDFA-L3/179  "IFC_Line01_Curv"
  Data Type Conversion19/1 -> SDFA-L3/168  "IFC_obj_LengthStdDev"
  Data Type Conversion239/1 -> SDFA-L3/218  "IFC_Line04_Curv"
  Data Type Conversion13/1 -> SDFA-L3/127  "IFC_State"
  Ground32/1 -> SDFA-L3/251  "FS_Out_Of_Calib"
  Subsystem212/1(obj_PhiLeft) -> Data Type Conversion38/1
  Data Type Conversion256/1 -> SDFA-L3/103  "AbsoluteLatVelo"
  Data Type Conversion57/1 -> SDFA-L3/181  "IFC_Line01_Dy"
  Data Type Conversion71/1 -> SDFA-L3/119  "ReferencePoint"
  Data Type Conversion242/1 -> SDFA-L3/221  "IFC_Line04_ExistProb"
  Data Type Conversion251/1 -> SDFA-L3/229  "IFC_Line04_LineWidth"
  Ground57/1 -> SDFA-L3/129  "FS_Sun_Ray_0"
  Read CM Dict12/1 -> Data Type Conversion59/1
  Subsystem190/1(obj_TTIPCSTD) -> Data Type Conversion21/1
  Subsystem218/1(obj_Height) -> Data Type Conversion45/1
  Data Type Conversion50/1 -> SDFA-L3/136  "IFC_obj_Type"
  Subsystem228/1(obj_Type) -> Data Type Conversion50/1
  Subsystem199/1(obj_Rel_VySTD) -> Data Type Conversion30/1
  Data Type Conversion64/1 -> SDFA-L3/188  "IFC_Line01_DxStart"
  Read CM Dict34/1 -> Data Type Conversion221/1
  Subsystem178/1(AbsLatAccSTD) -> Data Type Conversion9/1
  Subsystem149/1(obj_ExistProb) -> Data Type Conversion213/1
  Ground52/1 -> Data Type Conversion72/1
  Ground3/1 -> Data Type Conversion261/1
  Read CM Dict22/1 -> Data Type Conversion211/1
  Subsystem220/1(obj_Length) -> Data Type Conversion47/1
  Read CM Dict44/1 -> Data Type Conversion232/1
  Data Type Conversion4/1 -> SDFA-L3/91  "LongDistanceSTD"
  Ground59/1 -> SDFA-L3/131  "FS_Rain"
  Subsystem185/1(obj_WidthSTD) -> Data Type Conversion16/1
  Read CM Dict36/1 -> Data Type Conversion223/1
  Data Type Conversion237/1 -> SDFA-L3/216  "IFC_Line03_LineWidth"
  Data Type Conversion23/1 -> SDFA-L3/145  "IFC_obj_abs_Ax"
  Data Type Conversion80/1 -> SDFA-L3/142  "IFC_obj_Rel_VxStdDevValid"
  Data Type Conversion65/1 -> SDFA-L3/189  "IFC_Line01_DxEnd"
  Data Type Conversion43/1 -> SDFA-L3/113  "Widh"
  Subsystem206/1(Latdistance) -> Data Type Conversion3/1
  Data Type Conversion30/1 -> SDFA-L3/143  "IFC_obj_Rel_VyStdDev"
  Subsystem204/1(obj_abs_Ay) -> Data Type Conversion33/1
  Data Type Conversion255/1 -> SDFA-L3/105  "AbsoluteLatAcc"
  Data Type Conversion235/1 -> SDFA-L3/138  "IFC_obj_VxValid"
  Read CM Dict49/1 -> Data Type Conversion238/1
  Data Type Conversion211/1 -> SDFA-L3/193  "IFC_Line02_HeadingAngle"
  Subsystem201/1(AbsoluteLatAcc) -> Data Type Conversion255/1
  Read CM Dict20/1 -> Data Type Conversion67/1
  Data Type Conversion250/1 -> SDFA-L3/228  "IFC_Line04_DxEnd"
  Ground4/1 -> SDFA-L3/231  "IFC_Roaddge01_MessureType"
  Data Type  Conversion1/1 -> SDFA-L3/83  "SWINve_g_ESC_YawRate"
  Data Type Conversion67/1 -> SDFA-L3/191  "IFC_Line02_CurvChange"
  Subsystem4/1(Out1) -> Data Type Conversion69/1
  Data Type  Conversion6/1 -> SDFA-L3/85  "SWINve_g_ESC_LongitudinalAccelaration"
  Data Type  Conversion2/1 -> SDFA-L3/84  "SWINve_g_SAS_SteeringAngle"
  Data Type Conversion85/1 -> SDFA-L3/81  "system_clock"
  Data Type Conversion118/1 -> SDFA-L3/259  "CorrCoeff_y_vy"
  Data Type Conversion249/1 -> SDFA-L3/227  "IFC_Line04_DxStart"
  Data Type Conversion53/1 -> SDFA-L3/178  "IFC_Line01_CurvChange"
  Subsystem179/1(LengthSTD) -> Data Type Conversion10/1
  Data Type Conversion51/1 -> SDFA-L3/175  "IFC_obj_TTIPC"
  Read CM Dict26/1 -> Gain10/1
  Read CM Dict41/1 -> Data Type Conversion229/1
  Data Type Conversion254/1 -> SDFA-L3/109  "ClassType"
  Ground25/1 -> SDFA-L3/249  "IFC_Roaddge02_LineID"
  Ground37/1 -> SDFA-L3/256  "FS_Full_Windshield_0"
  Data Type Conversion129/1 -> SDFA-L3/261  "CorrCoeff_x_vy"
  Ground39/1 -> SDFA-L3/257  "FS_Out_Of_Focus_0"
  Constant3/1 -> Data Type Conversion129/1
  Subsystem20/1(Yaw_speed) -> Data Type  Conversion1/1  "Yaw_speed"
  Subsystem40/1(TimeStamp) -> Data Type Conversion98/1
  Ground36/1 -> SDFA-L3/255  "FS_Full_Blockage_0"
  Read CM Dict48/1 -> Data Type Conversion237/1
  Data Type Conversion128/1 -> SDFA-L3/260  "CorrCoeff_y_vx"
  Constant1/1 -> Data Type Conversion118/1
  Data Type Conversion69/1 -> SDFA-L3/250  "camera_timestamp"
  Read CM Dict37/1 -> Data Type Conversion225/1
  Data Type Conversion228/1 -> SDFA-L3/208  "IFC_Line03_ExistProb"
  Ground34/1 -> SDFA-L3/253  "FS_Blur_Image_0"
  Data Type Conversion60/1 -> SDFA-L3/133  "IFC_ObjHdr_ObjCount"
  Data Type Conversion17/1 -> SDFA-L3/162  "IFC_obj_angle_rate_StdDev"
  Constant9/1 -> Data Type Conversion265/1
  Subsystem191/1(obj_PhiBottomSTD) -> Data Type Conversion22/1
  Data Type Conversion32/1 -> SDFA-L3/123  "MeasurementStatus"
  Data Type Conversion/1 -> SDFA-L3/258  "CorrCoeff_x_vx"
  Data Type Conversion98/1 -> SDFA-L3/87  "TimeStamp"
  Subsystem211/1(Widh) -> Data Type Conversion43/1
  Data Type Conversion44/1 -> SDFA-L3/163  "IFC_obj_Width"
  Data Type Conversion45/1 -> SDFA-L3/165  "IFC_obj_Height"
  Data Type Conversion214/1 -> SDFA-L3/195  "IFC_Line02_ExistProb"
  Subsystem171/1(obj_Rel_VxValid) -> Data Type Conversion235/1
  Data Type Conversion213/1 -> SDFA-L3/134  "IFC_obj_ExistProb"
  Subsystem210/1(obj_Dy) -> Data Type Conversion37/1
  Lateral_acceleration1/1 -> Data Type  Conversion3/1  "Lateral_acceleration"
  Read CM Dict2/1 -> Data Type Conversion13/1  "IFCState"
  Data Type Conversion6/1 -> SDFA-L3/100  "AbsLongVeloSTD"
  Subsystem208/1(obj_Dx) -> Data Type Conversion35/1
  Subsystem197/1(obj_abs_AySTD) -> Data Type Conversion28/1
  Subsystem216/1(obj_Width) -> Data Type Conversion44/1
  Read CM Dict55/1 -> Data Type Conversion244/1
  Read CM Dict62/1 -> Data Type Conversion60/1
  Read CM Dict53/1 -> Data Type Conversion242/1
  Read CM Dict27/1 -> Saturation3/1  "Steering_wheel_angle"
  Data Type Conversion245/1 -> SDFA-L3/224  "IFC_Line04_LineID"
  Data Type Conversion231/1 -> SDFA-L3/211  "IFC_Line03_LineID"
  Subsystem221/1(MovementStatus) -> Data Type Conversion34/1
  Subsystem225/1(ExistenceProb) -> Data Type Conversion257/1
  Subsystem/1(Out1) -> Data Type Conversion85/1
  Subsystem2/1(ObjectAge) -> Data Type Conversion70/1
  Subsystem3/1(ReferencePoint) -> Data Type Conversion71/1
  Data Type Conversion72/1 -> SDFA-L3/94  "DistanceCovariance"
  Subsystem5/1(obj_BrakeLight) -> Data Type Conversion73/1
  Subsystem6/1(obj_HeadOrientation) -> Data Type Conversion74/1
  Data Type Conversion74/1 -> SDFA-L3/173  "IFC_obj_HeadOrientation"
  Subsystem7/1(obj_DirIndicator) -> Data Type Conversion75/1
  Subsystem8/1(obj_angle_rate) -> Data Type Conversion76/1
  Subsystem9/1(obj_angle_3D) -> Data Type Conversion77/1
  Subsystem10/1(obj_PhiBottom) -> Data Type Conversion78/1
  Subsystem11/1(obj_Rel_VyStdDevValid) -> Data Type Conversion79/1
  Subsystem12/1(obj_Rel_VxStdDevValid) -> Data Type Conversion80/1
  Subsystem14/1(RadarCrossSection) -> Data Type Conversion81/1
  Constant4/1 -> Data Type Conversion/1
  Data Type Conversion42/1 -> SDFA-L3/263
  Constant5/1 -> Data Type Conversion42/1
  Data Type Conversion82/1 -> SDFA-L3/266
  Constant6/1 -> Data Type Conversion82/1
  Constant7/1 -> Data Type Conversion83/1
  Data Type Conversion83/1 -> SDFA-L3/268
  Constant8/1 -> Data Type Conversion84/1
  Constant10/1 -> Data Type Conversion86/1
  Data Type Conversion84/1 -> SDFA-L3/269
  Data Type Conversion86/1 -> SDFA-L3/270
  Data Type Conversion89/1 -> SDFA-L3/273
  Data Type Conversion88/1 -> SDFA-L3/272
  Constant11/1 -> Data Type Conversion89/1
  Constant13/1 -> Data Type Conversion88/1
  Data Type Conversion87/1 -> SDFA-L3/271
  Constant12/1 -> Data Type Conversion87/1
  Constant16/1 -> Data Type Conversion93/1
  Data Type Conversion93/1 -> SDFA-L3/277
  Constant17/1 -> Data Type Conversion94/1
  Data Type Conversion94/1 -> SDFA-L3/278
  Data Type Conversion92/1 -> SDFA-L3/276
  Data Type Conversion91/1 -> SDFA-L3/275
  Constant14/1 -> Data Type Conversion92/1
  Constant19/1 -> Data Type Conversion91/1
  Data Type Conversion90/1 -> SDFA-L3/274
  Constant18/1 -> Data Type Conversion90/1
  SDFA-L3/106 -> BusCreator3/106  "SDFAve_g_Rrg_VIEW_RANGE_end"
  SDFA-L3/7 -> BusCreator3/7  "SDFAve_g_fusion_time_stamp"
  SDFA-L3/8 -> BusCreator3/8  "SDFAve_d_obj_Num"
  SDFA-L3/9 -> BusCreator3/9  "SDFAva_d_obj_id"
  SDFA-L3/10 -> BusCreator3/10  "SDFAva_g_obj_pos_x"
  SDFA-L3/11 -> BusCreator3/11  "SDFAva_g_obj_pos_y"
  SDFA-L3/12 -> BusCreator3/12  "SDFAva_g_obj_vel_x"
  SDFA-L3/13 -> BusCreator3/13  "SDFAva_g_obj_vel_y"
  SDFA-L3/14 -> BusCreator3/14  "SDFAva_g_obj_acc_x"
  SDFA-L3/15 -> BusCreator3/15  "SDFAva_g_obj_acc_y"
  SDFA-L3/16 -> BusCreator3/16  "SDFAva_g_obj_pos_var_x"
  SDFA-L3/17 -> BusCreator3/17  "SDFAva_g_obj_pos_var_y"
  SDFA-L3/18 -> BusCreator3/18  "SDFAva_g_obj_pos_var_xy"
  SDFA-L3/19 -> BusCreator3/19  "SDFAva_g_obj_width"
  SDFA-L3/20 -> BusCreator3/20  "SDFAva_g_obj_length"
  SDFA-L3/21 -> BusCreator3/21  "SDFAva_d_obj_class"
  SDFA-L3/22 -> BusCreator3/22  "SDFAva_d_obj_lane"
  SDFA-L3/23 -> BusCreator3/23  "SDFAva_y_obj_status"
  SDFA-L3/24 -> BusCreator3/24  "SDFAve_g_obj_age"
  SDFA-L3/25 -> BusCreator3/25  "SDFAva_y_obj_TurnLight"
  SDFA-L3/26 -> BusCreator3/26  "SDFAva_d_obj_BrakeLight"
  SDFA-L3/27 -> BusCreator3/27  "SDFAva_y_obj_MotionStatus"
  SDFA-L3/28 -> BusCreator3/28  "SDFAve_y_ISAValue"
  SDFA-L3/29 -> BusCreator3/29  "SDFAve_y_TSR_Sign_Type"
  SDFA-L3/30 -> BusCreator3/30  "SDFAve_g_CameraSignalFault"
  SDFA-L3/31 -> BusCreator3/31  "SDFAve_y_Road_TYPE"
  SDFA-L3/32 -> BusCreator3/32  "SDFAve_g_L0_C0_COEF"
  SDFA-L3/33 -> BusCreator3/33  "SDFAve_g_L0_C1_COEF"
  SDFA-L3/34 -> BusCreator3/34  "SDFAve_g_L0_C2_COEF"
  SDFA-L3/35 -> BusCreator3/35  "SDFAve_g_L0_C3_COEF"
  SDFA-L3/36 -> BusCreator3/36  "SDFAve_g_L0_VIEW_RANGE"
  SDFA-L3/37 -> BusCreator3/37  "SDFAve_g_L0_DETECT_QUALITY"
  SDFA-L3/38 -> BusCreator3/38  "SDFAve_d_L0_LINE_TYPE"
  SDFA-L3/39 -> BusCreator3/39  "SDFAve_g_L0_MARK_WIDTH"
  SDFA-L3/40 -> BusCreator3/40  "SDFAve_g_R0_C0_COEF"
  SDFA-L3/41 -> BusCreator3/41  "SDFAve_g_R0_C1_COEF"
  SDFA-L3/42 -> BusCreator3/42  "SDFAve_g_R0_C2_COEF"
  SDFA-L3/43 -> BusCreator3/43  "SDFAve_g_R0_C3_COEF"
  SDFA-L3/44 -> BusCreator3/44  "SDFAve_g_R0_VIEW_RANGE"
  SDFA-L3/45 -> BusCreator3/45  "SDFAve_y_R0_DETECT_QUALITY"
  SDFA-L3/46 -> BusCreator3/46  "SDFAve_d_R0_LINE_TYPE"
  SDFA-L3/47 -> BusCreator3/47  "SDFAve_g_R0_MARK_WIDTH"
  SDFA-L3/48 -> BusCreator3/48  "SDFAve_g_R0_VIEW_RANGE"
  SDFA-L3/49 -> BusCreator3/49  "SDFAve_g_L1_C1_COEF"
  SDFA-L3/50 -> BusCreator3/50  "SDFAve_g_L1_C2_COEF"
  SDFA-L3/51 -> BusCreator3/51  "SDFAve_g_L1_C3_COEF"
  SDFA-L3/52 -> BusCreator3/52  "SDFAve_g_L1_VIEW_RANGE"
  SDFA-L3/53 -> BusCreator3/53  "SDFAve_y_L1_DETECT_QUALITY"
  SDFA-L3/54 -> BusCreator3/54  "SDFAve_d_L1_LINE_TYPE"
  SDFA-L3/55 -> BusCreator3/55  "SDFAve_g_L1_MARK_WIDTH"
  SDFA-L3/56 -> BusCreator3/56  "SDFAve_g_R1_C0_COEF"
  SDFA-L3/57 -> BusCreator3/57  "SDFAve_g_R1_C1_COEF"
  SDFA-L3/58 -> BusCreator3/58  "SDFAve_g_R1_C2_COEF"
  SDFA-L3/59 -> BusCreator3/59  "SDFAve_g_R1_C3_COEF"
  SDFA-L3/60 -> BusCreator3/60  "SDFAve_g_R1_VIEW_RANGE"
  SDFA-L3/61 -> BusCreator3/61  "SDFAve_y_R1_DETECT_QUALITY"
  SDFA-L3/62 -> BusCreator3/62  "SDFAve_d_R1_LINE_TYPE"
  SDFA-L3/63 -> BusCreator3/63  "SDFAve_g_R1_MARK_WIDTH"
  SDFA-L3/64 -> BusCreator3/64  "SDFAve_g_L0_C0_BACK_COEF"
  SDFA-L3/65 -> BusCreator3/65  "SDFAve_g_L0_C1_BACK_COEF"
  SDFA-L3/66 -> BusCreator3/66  "SDFAve_g_L0_C2_BACK_COEF"
  SDFA-L3/67 -> BusCreator3/67  "SDFAve_g_L0_C3_BACK_COEF"
  SDFA-L3/68 -> BusCreator3/68  "SDFAve_g_L0_BACK_RANGE"
  SDFA-L3/69 -> BusCreator3/69  "SDFAve_g_R0_C0_BACK_COEF"
  SDFA-L3/70 -> BusCreator3/70  "SDFAve_g_R0_C1_BACK_COEF"
  SDFA-L3/71 -> BusCreator3/71  "SDFAve_g_L0_C0_BACK_COEF"
  SDFA-L3/72 -> BusCreator3/72  "SDFAve_g_R0_C3_BACK_COEF"
  SDFA-L3/73 -> BusCreator3/73  "SDFAve_g_R0_BACK_RANGE"
  SDFA-L3/74 -> BusCreator3/74  "SDFAve_g_L1_C0_BACK_COEF"
  SDFA-L3/75 -> BusCreator3/75  "SDFAve_g_L1_C1_BACK_COEF"
  SDFA-L3/76 -> BusCreator3/76  "SDFAve_g_L1_C2_BACK_COEF"
  SDFA-L3/77 -> BusCreator3/77  "SDFAve_g_L1_C3_BACK_COEF"
  SDFA-L3/78 -> BusCreator3/78  "SDFAve_g_L1_BACK_RANGE"
  SDFA-L3/79 -> BusCreator3/79  "SDFAve_g_R1_C0_BACK_COEF"
  SDFA-L3/80 -> BusCreator3/80  "SDFAve_g_R1_C1_BACK_COEF"
  SDFA-L3/81 -> BusCreator3/81  "SDFAve_g_R1_C2_BACK_COEF"
  SDFA-L3/82 -> BusCreator3/82  "SDFAve_g_R1_C3_BACK_COEF"
  SDFA-L3/83 -> BusCreator3/83  "SDFAve_g_R1_BACK_RANGE"
  SDFA-L3/84 -> BusCreator3/84  "SDFAve_y_ADAS_IHBC_Fuction_Status"
  SDFA-L3/85 -> BusCreator3/85  "SDFAve_y_ADAS_IHBC_High_Beam_Req"
  SDFA-L3/86 -> BusCreator3/86  "SDFAve_y_ISASignType"
  SDFA-L3/87 -> BusCreator3/87  "SDFAve_y_ISAStatus"
  SDFA-L3/88 -> BusCreator3/88  "SDFAve_y_ISAPopupMessage"
  SDFA-L3/89 -> BusCreator3/89  "SDFAve_y_Radar_State"
  SDFA-L3/90 -> BusCreator3/90  "SDFAve_y_OperatinfStatus"
  SDFA-L3/91 -> BusCreator3/91  "SDFAve_d_CorRadarDTC"
  SDFA-L3/92 -> BusCreator3/92  "SDFAve_g_ForeRadarDTC"
  SDFA-L3/93 -> BusCreator3/93  "SDFAve_g_CameraDTC"
  SDFA-L3/94 -> BusCreator3/94  "SDFAve_y_Radar_FaultBitSetting_Signal"
  SDFA-L3/95 -> BusCreator3/95  "SDFAve_g_Lrg_C0_BACK_COEF"
  SDFA-L3/96 -> BusCreator3/96  "SDFAve_g_Lrg_C1_BACK_COEF"
  SDFA-L3/97 -> BusCreator3/97  "SDFAve_g_Lrg_C2_BACK_COEF"
  SDFA-L3/98 -> BusCreator3/98  "SDFAve_g_Lrg_C3_BACK_COEF"
  SDFA-L3/99 -> BusCreator3/99  "SDFAve_g_Lrg_VIEW_RANGE_start"
  SDFA-L3/100 -> BusCreator3/100  "SDFAve_g_Lrg_VIEW_RANGE_end"
  SDFA-L3/101 -> BusCreator3/101  "SDFAve_g_Rrg_C0_BACK_COEF"
  SDFA-L3/102 -> BusCreator3/102  "SDFAve_g_Rrg_C1_BACK_COEF"
  SDFA-L3/103 -> BusCreator3/103  "SDFAve_g_Rrg_C2_BACK_COEF"
  SDFA-L3/104 -> BusCreator3/104  "SDFAve_g_Rrg_C3_BACK_COEF"
  SDFA-L3/105 -> BusCreator3/105  "SDFAve_g_Rrg_VIEW_RANGE_start"
  SDFA-L3/107 -> BusCreator3/107  "SDFAve_y_Rrg_DETECT_QUALITY"
  SDFA-L3/108 -> BusCreator3/108  "SDFAve_y_Rrg_LINE_TYPE"
  SDFA-L3/109 -> BusCreator3/109  "SDFAve_y_Lrg_DETECT_QUALITY"
  SDFA-L3/110 -> BusCreator3/110  "SDFAve_y_Lrg_LINE_TYPE"
  [ICAMode] -> SDFA-L3/311
